simulink model "Driving_dynamics_model"  (R2022b)
settings: Solver=VariableStepAuto  StartTime=0.0  StopTime=10.0  RelTol=1e-3
values from neighbouring files (symbols this model uses):
  A = 1.25    [Longitudinal_braking_parameters.m]    (also in Longitudinal_driving_parameters.m)
  a = 1.8    [Longitudinal_braking_parameters.m]    (also in Longitudinal_driving_parameters.m)
  a1 = -1e-5    (= -1e-05)    [Longitudinal_braking_parameters.m]    (also in Longitudinal_driving_parameters.m; Pacejka_lateral_parameters.m)
  a2 = 1.25    [Longitudinal_braking_parameters.m]    (also in Longitudinal_driving_parameters.m; Pacejka_lateral_parameters.m)
  B = 4.1576    [Longitudinal_braking_parameters.m]    (also in Longitudinal_driving_parameters.m = 5.7507; Pacejka_lateral_parameters.m = 0.1453)
  C = 1.7180    (= 1.718)    [Longitudinal_braking_parameters.m]    (also in Longitudinal_driving_parameters.m = 1.2421; Pacejka_lateral_parameters.m = 1.5511)
  cd = 0.4    [Longitudinal_braking_parameters.m]    (also in Longitudinal_driving_parameters.m)
  cz = 1    [Longitudinal_braking_parameters.m]    (also in Longitudinal_driving_parameters.m)
  enginemap = [-0.15, 0.23, 0.60, 0.68, 0.80 ... (first row only)    [Longitudinal_driving_parameters.m]
  enginerpm = linspace(1000,15000,15)'    [Longitudinal_driving_parameters.m]
  g = 9.81    [Longitudinal_braking_parameters.m]    (also in Longitudinal_driving_parameters.m; Quarter_car_model_parameters.m)
  h = 0.2    [Longitudinal_braking_parameters.m]    (also in Longitudinal_driving_parameters.m)
  Iwheel = 0.9    [Longitudinal_braking_parameters.m]    (also in Longitudinal_driving_parameters.m)
  L = 3.5    [Longitudinal_braking_parameters.m]    (also in Longitudinal_driving_parameters.m)
  m = 850    [Longitudinal_braking_parameters.m]    (also in Longitudinal_driving_parameters.m)
  r = 0.375    [Longitudinal_braking_parameters.m]    (also in Longitudinal_driving_parameters.m)
  rho = 1.225    [Longitudinal_braking_parameters.m]    (also in Longitudinal_driving_parameters.m)
  Tengmax = 250    [Longitudinal_driving_parameters.m]
  throttlepos = [0, 0.25, 0.5, 0.75, 1]'    [Longitudinal_driving_parameters.m]
settings Model: Creator=webstert  LastModifiedBy=webstert

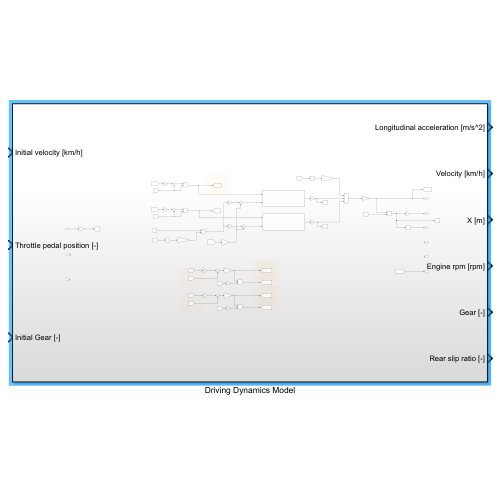
[thumbnail: Simulink's stored preview of the top-level diagram]
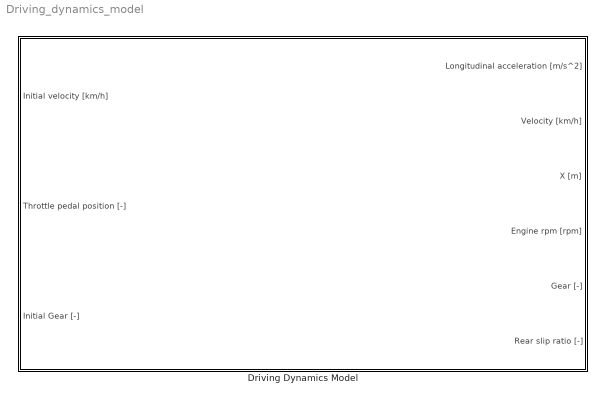
== system Driving_dynamics_model ==
  Driving Dynamics Model : Subsystem

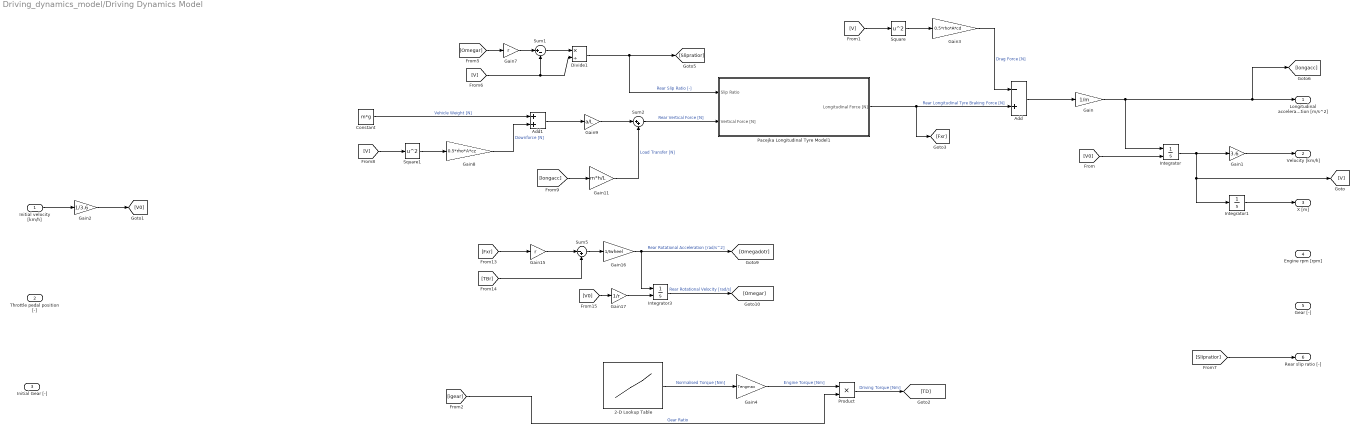
== system Driving_dynamics_model/Driving Dynamics Model ==
  Initial velocity [km/h] : Inport
  Throttle pedal position [-] : Inport  Port=2
  Initial Gear [-] : Inport  Port=3
  2-D Lookup Table : Lookup_n-D  BreakpointsForDimension1=enginerpm  BreakpointsForDimension2=throttlepos  Table=enginemap  InternalRulePriority=Speed  RndMeth=Simplest
      settings: InputPortMap=u0,u1
  Add : Sum  Inputs=-+
  Add1 : Sum
  Constant : Constant  Value=m*g
  Divide1 : Product  Inputs=*/
  Gain : Gain  Gain=1/m
  Gain1 : Gain  Gain=3.6
  Gain11 : Gain  Gain=m*h/L
  Gain15 : Gain  Gain=r
  Gain16 : Gain  Gain=1/Iwheel
  Gain17 : Gain  Gain=1/r
  Gain2 : Gain  Gain=1/3.6
  Gain3 : Gain  Gain=0.5*rho*A*cd
  Gain4 : Gain  Gain=Tengmax
  Gain7 : Gain  Gain=r
  Gain8 : Gain  Gain=0.5*rho*A*cz
  Gain9 : Gain  Gain=a/L
  Integrator : Integrator  InitialConditionSource=external
  Integrator1 : Integrator
  Integrator3 : Integrator  InitialConditionSource=external
  Pacejka Longitudinal Tyre Model1 : Subsystem
  Product : Product
  Square : Math  Operator=square
  Square1 : Math  Operator=square
  Sum1 : Sum  Inputs=|+-
  Sum2 : Sum  Inputs=|++
  Sum5 : Sum  Inputs=|-+
  Longitudinal acceleration [m/s^2] : Outport
  Velocity [km/h] : Outport  Port=2
  X [m] : Outport  Port=3
  Engine rpm [rpm] : Outport  Port=4
  Gear [-] : Outport  Port=5
  Rear slip ratio [-] : Outport  Port=6
  wires:
  Add/1 -> Gain/1
  Sum5/1 -> Gain16/1
  Gain15/1 -> Sum5/1
  Gain17/1 -> Integrator3/2
  [V] -> Square/1
  [longacc] -> Gain11/1
  Integrator3/1 -> [Omegar]  "Rear Rotational Velocity [rad/s]"
  [TBr] -> Sum5/2
  Gain11/1 -> Sum2/2  "Load Transfer [N]"
  [V0] -> Gain17/1
  [Fxr] -> Gain15/1
  Add1/1 -> Gain9/1
  Gain1/1 -> Velocity [km/h]/1
  Sum2/1 -> Pacejka Longitudinal Tyre Model1/2(Vertical Force [N])  "Rear Vertical Force [N]"
  Sum1/1 -> Divide1/1
  [V] -> Square1/1
  [Omegar] -> Gain7/1
  Gain8/1 -> Add1/2  "Downforce [N]"
  Divide1/1 -> Pacejka Longitudinal Tyre Model1/1(Slip Ratio), [Slipratior]  "Rear Slip Ratio [-]"
  Integrator1/1 -> X [m]/1
  [V0] -> Integrator/2
  Pacejka Longitudinal Tyre Model1/1(Longitudinal Force [N]) -> [Fxr], Add/2  "Rear Longitudinal Tyre Braking Force [N]"
  Gain16/1 -> [Omegadotr], Integrator3/1  "Rear Rotational Acceleration [rad/s^2]"
  [Slipratior] -> Rear slip ratio [-]/1
  Square1/1 -> Gain8/1
  Square/1 -> Gain3/1
  Initial velocity [km/h]/1 -> Gain2/1
  Gain9/1 -> Sum2/1
  Integrator/1 -> Gain1/1, [V], Integrator1/1
  Gain2/1 -> [V0]
  Constant/1 -> Add1/1  "Vehicle Weight [N]"
  Gain7/1 -> Sum1/1
  Gain3/1 -> Add/1  "Drag Force [N]"
  [V] -> Divide1/2, Sum1/2
  Gain/1 -> Integrator/1, [longacc], Longitudinal acceleration [m/s^2]/1
  2-D Lookup Table/1 -> Gain4/1  "Normalised Torque [Nm]"
  Gain4/1 -> Product/1  "Engine Torque [Nm]"
  [igear] -> Product/2  "Gear Ratio"
  Product/1 -> [TD]  "Driving Torque [Nm]"

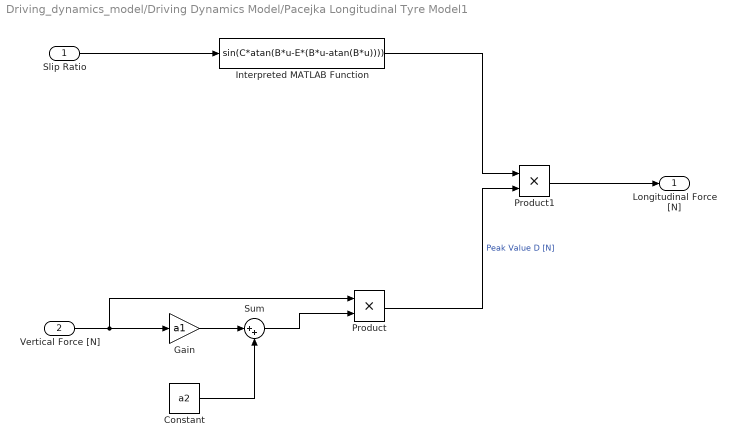
== system Driving_dynamics_model/Driving Dynamics Model/Pacejka Longitudinal Tyre Model1 ==
  Slip Ratio : Inport
  Vertical Force [N] : Inport  Port=2
  Constant : Constant  Value=a2
  Gain : Gain  Gain=a1
  Interpreted MATLAB Function : MATLABFcn  MATLABFcn=sin(C*atan(B*u-E*(B*u-atan(B*u))))
  Product : Product
  Product1 : Product
  Sum : Sum  Inputs=|++
  Longitudinal Force [N] : Outport
  wires:
  Product1/1 -> Longitudinal Force [N]/1
  Interpreted MATLAB Function/1 -> Product1/1
  Slip Ratio/1 -> Interpreted MATLAB Function/1
  Product/1 -> Product1/2  "Peak Value D [N]"
  Sum/1 -> Product/2
  Gain/1 -> Sum/1
  Constant/1 -> Sum/2
  Vertical Force [N]/1 -> Gain/1, Product/1
